simulink model "ekf9mlf_example"  (R2014a)
settings: Solver=FixedStepDiscrete  StartTime=0  StopTime=200  RelTol=1e-3
settings Model: Creator=gcampa  LastModifiedBy=gcampa
settings DataIOCC: LimitDataPoints=off  SignalLoggingSaveFormat=ModelDataLogs  SaveOutput=off  SaveTime=off
settings OptimizationCC: BlockReduction=off  BooleanDataType=off  ExpressionDepthLimit=2147483647  InitFltsAndDblsToZero=on
settings DebuggingCC: SaveWithParameterizedLinksMsg=none  UnderspecifiedInitializationDetection=Classic  SignalResolutionControl=TryResolveAllWithWarning  SolverPrmCheckMsg=none  MultiTaskDSMMsg=warning  MultiTaskCondExecSysMsg=none  FcnCallInpInsideContextMsg=UseLocalSettings  StateNameClashWarn=warning
settings HardwareCC: TargetLongLongMode=on  TargetIntDivRoundTo=Zero  TargetEndianess=LittleEndian  TargetHWDeviceType=MATLAB Host  ProdEqTarget=off
settings RTWCC: IncludeERTFirstTime=on  RTWCompilerOptimization=On
settings GRTTargetCC: TargetFcnLib=ansi_tfl_tmw.mat  CombineOutputUpdateFcns=off  GRTInterface=on

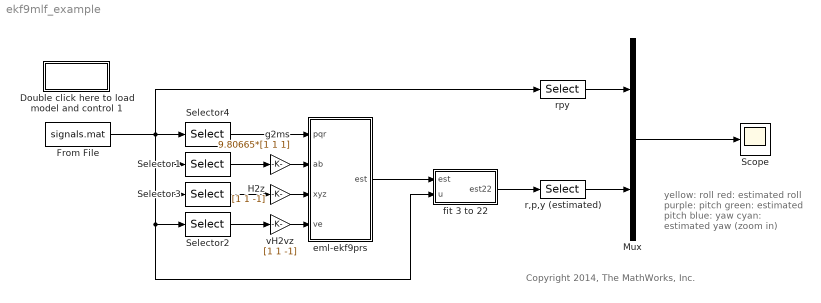
== system ekf9mlf_example ==
  note: yellow: roll
      | red: estimated roll
      | purple: pitch
      | green: estimated pitch
      | blue: yaw
      | cyan: estimated yaw
      | (zoom in)
  note: Copyright 2014, The MathWorks, Inc.
  Double click here to load model and control 1 : Subsystem
      mask Display: disp('Measured \nSignals')
  From File : FromFile  FileName=signals.mat  SampleTime=0.05
  H2z : Gain  Gain=[1 1 -1]  SaturateOnIntegerOverflow=on  OutDataTypeStr=Inherit: Same as input  ParamDataTypeStr=Inherit: Same as input
  Mux : Mux  Inputs=[3 3]
  Scope : Scope
  Selector1 : Selector  InputPortWidth=22  Indices=16:18
  Selector2 : Selector  InputPortWidth=22  Indices=13:15
  Selector3 : Selector  InputPortWidth=22  Indices=13:15
  Selector4 : Selector  InputPortWidth=22  Indices=[4:6]
  eml-ekf9prs : MATLAB Function  TreatAsAtomicUnit=on
  fit 3 to 22 : Subsystem
  g2ms : Gain  Gain=9.80665*[1 1 1]  SaturateOnIntegerOverflow=on  OutDataTypeStr=Inherit: Same as input  ParamDataTypeStr=Inherit: Same as input
  r,p,y (estimated) : Selector  InputPortWidth=22  Indices=[9 8 7]
  rpy : Selector  InputPortWidth=22  Indices=[9 8 7]
  vH2vz : Gain  Gain=[1 1 -1]  SaturateOnIntegerOverflow=on  OutDataTypeStr=Inherit: Same as input  ParamDataTypeStr=Inherit: Same as input
  wires:
  fit 3 to 22/1(est22) -> r,p,y (estimated)/1
  Selector3/1 -> H2z/1
  Selector1/1 -> g2ms/1
  g2ms/1 -> eml-ekf9prs/2(ab)
  Selector4/1 -> eml-ekf9prs/1(pqr)
  From File/1 -> rpy/1, Selector3/1, Selector2/1, fit 3 to 22/2(u), Selector1/1, Selector4/1
  eml-ekf9prs/1(est) -> fit 3 to 22/1(est)
  H2z/1 -> eml-ekf9prs/3(xyz)
  vH2vz/1 -> eml-ekf9prs/4(ve)
  Selector2/1 -> vH2vz/1
  rpy/1 -> Mux/1
  r,p,y (estimated)/1 -> Mux/2
  Mux/1 -> Scope/1

== system ekf9mlf_example/Double click here to load model and control 1 ==
  note: More information on the aircraft model and controllers can be found here:
      | http://www.mathworks.com/matlabcentral/fileexchange/3019-airlib
  note: An aircraft model in closed loop with an inner and outer loop feedback
      | linearization control system was used to generate attitude (roll, pitch and yaw)
      | as well as all the other relevant signals
  note: x:
      |
      | 01    v           (m/s)
      | 02    alpha    (rad)
      | 03    beta      (rad)
      | 04    p           (rad/s)
      | 05    q           (rad/s)
      | 06    r            (rad/s)
      | 07    psi         (rad)
      | 08    theta     (rad)
      | 09    phi        (rad)
      | 10    x           (m)
      | 11    y           (m)
      | 12    H          (m)
      |
      | x_dot (NED earth frame):
      |
      | 13    x_dot     (m/s)
      | 14    y_dot     (m/s)
      | 15    z_dot     (m/s)
      |
      | accelerations:
      |
      | 16    Ax     (g)
      | 17    Ay     (g)
      | 18    Az     (g)
      |
      | controls:
      |
      | 19    delta elevators    (rad)
      | 20    delta ailerons      (rad)
      | 21    delta rudder        (rad)
      | 22    throttle             (Fx, N)

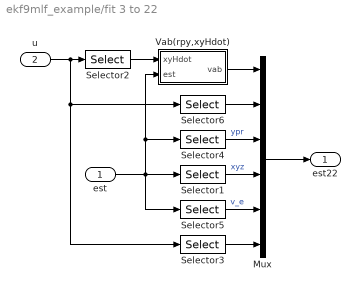
== system ekf9mlf_example/fit 3 to 22 ==
  est : Inport
  u : Inport  Port=2
  Mux : Mux  Inputs=[3 3 3 3 3 7]
  Selector1 : Selector  InputPortWidth=9  Indices=1:3
  Selector2 : Selector  InputPortWidth=22  Indices=13:15
  Selector3 : Selector  InputPortWidth=22  Indices=16:22
  Selector4 : Selector  InputPortWidth=9  Indices=[9 8 7]
  Selector5 : Selector  InputPortWidth=9  Indices=4:6
  Selector6 : Selector  InputPortWidth=22  Indices=4:6
  Vab(rpy,xyHdot) : Subsystem
  est22 : Outport
  wires:
  Selector6/1 -> Mux/2
  Selector5/1 -> Mux/5  "v_e"
  Selector1/1 -> Mux/4  "xyz"
  Selector4/1 -> Mux/3  "ypr"
  Selector3/1 -> Mux/6
  Selector2/1 -> Vab(rpy,xyHdot)/1(xyHdot)
  Vab(rpy,xyHdot)/1(vab) -> Mux/1
  u/1 -> Selector6/1, Selector3/1, Selector2/1
  est/1 -> Selector5/1, Selector4/1, Vab(rpy,xyHdot)/2(est), Selector1/1
  Mux/1 -> est22/1

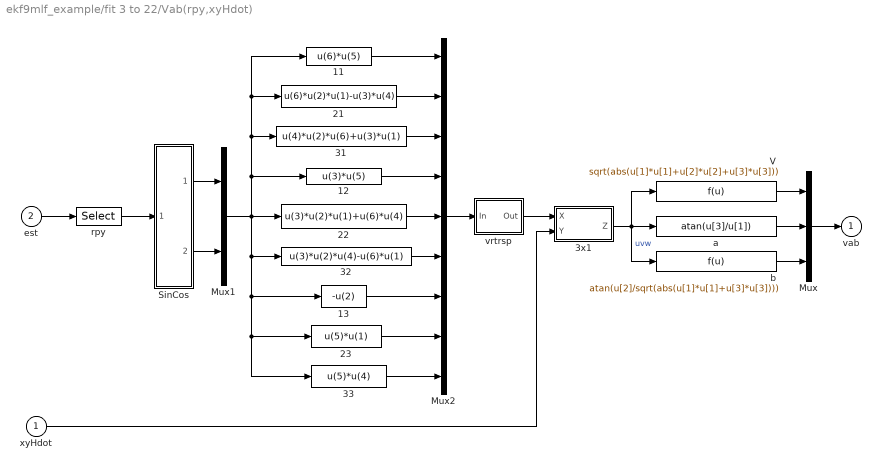
== system ekf9mlf_example/fit 3 to 22/Vab(rpy,xyHdot) ==
  xyHdot : Inport
  est : Inport  Port=2
  11 : Fcn  Expr=u(6)*u(5)
  12 : Fcn  Expr=u(3)*u(5)
  13 : Fcn  Expr=-u(2)
  21 : Fcn  Expr=u(6)*u(2)*u(1)-u(3)*u(4)
  22 : Fcn  Expr=u(3)*u(2)*u(1)+u(6)*u(4)
  23 : Fcn  Expr=u(5)*u(1)
  31 : Fcn  Expr=u(4)*u(2)*u(6)+u(3)*u(1)
  32 : Fcn  Expr=u(3)*u(2)*u(4)-u(6)*u(1)
  33 : Fcn  Expr=u(5)*u(4)
  3x1 : Subsystem  mask(3x3 Matrix Multiplication){}
      mask help:
      | Input 1   : elements of matrix X (3 by 3)
      |   Input 2   : elements of matrix Y (3 by 3)
      |   Output   : elements of matrix X*Y (3 by 3)
      mask Help:
      | <p>
      | Elements of input and output matrices are taken columnwise.
      | </p>
      mask Display: disp('Z=X*Y')
  Mux : Mux  Inputs=3
  Mux1 : Mux  Inputs=2
  Mux2 : Mux  Inputs=9
  SinCos : Subsystem  mask(SinCos){}
      mask help: Compute the sine and cosine of input, u. u is in radians.
      mask Help: web(asbhelp);
      mask Display:
      | port_label('output',1,'sin(u)','texmode','on');
      | port_label('output',2,'cos(u)','texmode','on');
  V : Fcn  Expr=sqrt(abs(u[1]*u[1]+u[2]*u[2]+u[3]*u[3]))
  a : Fcn  Expr=atan(u[3]/u[1])
  b : Fcn  Expr=atan(u[2]/sqrt(abs(u[1]*u[1]+u[3]*u[3])))
  rpy : Selector  InputPortWidth=9  Indices=7:9
  vrtrsp : Subsystem  mask(Simulink Matrix Library Block){dims=[3 3]}
      mask prompts: dims "[n m]"
      mask help:
      | Real Varying Matrix Transposition
      |   Input      : elements of matrix X (n by m)
      |   Output   : elements of matrix X' (m by n)
      mask Help:
      | <p>
      | Elements of input and output matrices are taken columnwise.
      | </p>
      | <p>
      | To use this block you should have the smxl library in your path.
      | </p>
      mask Display: disp('Y=X''')
  vab : Outport
  wires:
  rpy/1 -> SinCos/1(theta)
  vrtrsp/1(Out) -> 3x1/1(X)
  33/1 -> Mux2/9
  23/1 -> Mux2/8
  13/1 -> Mux2/7
  32/1 -> Mux2/6
  22/1 -> Mux2/5
  12/1 -> Mux2/4
  31/1 -> Mux2/3
  21/1 -> Mux2/2
  11/1 -> Mux2/1
  SinCos/1(sin(theta)) -> Mux1/1
  SinCos/2(cos(theta)) -> Mux1/2
  Mux1/1 -> 22/1, 11/1, 21/1, 31/1, 12/1, 32/1, 13/1, 23/1, 33/1
  Mux2/1 -> vrtrsp/1(In)
  xyHdot/1 -> 3x1/2(Y)
  b/1 -> Mux/3
  V/1 -> Mux/1
  a/1 -> Mux/2
  Mux/1 -> vab/1
  3x1/1(Z) -> b/1, a/1, V/1  "uvw"
  est/1 -> rpy/1

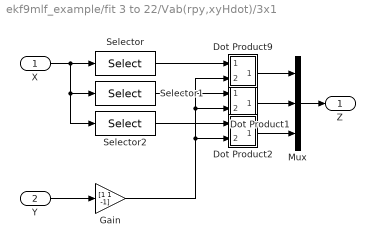
== system ekf9mlf_example/fit 3 to 22/Vab(rpy,xyHdot)/3x1 ==
  X : Inport
  Y : Inport  Port=2
  Dot Product1 : Subsystem  mask(Dot Product){}
      mask help:
      | Inner (dot) product.
      | y = sum(conj(u1).*u2). The operand u1 corresponds to the top (or left) input port.
      mask init:
      | t=(0:.1:2*pi)';
      | x=cos(t);
      | y=sin(t);
      | r=0.05;
      mask Help: Computes the inner (dot) product of the inputs: sum(u1.*u2).  The inputs are vectors of the same length. Output is a scalar.
      mask Display: patch([x*r+0.5],[y*r+0.5])
  Dot Product2 : Subsystem  mask(Dot Product){}
      mask help:
      | Inner (dot) product.
      | y = sum(conj(u1).*u2). The operand u1 corresponds to the top (or left) input port.
      mask init:
      | t=(0:.1:2*pi)';
      | x=cos(t);
      | y=sin(t);
      | r=0.05;
      mask Help: Computes the inner (dot) product of the inputs: sum(u1.*u2).  The inputs are vectors of the same length. Output is a scalar.
      mask Display: patch([x*r+0.5],[y*r+0.5])
  Dot Product9 : Subsystem  mask(Dot Product){}
      mask help:
      | Inner (dot) product.
      | y = sum(conj(u1).*u2). The operand u1 corresponds to the top (or left) input port.
      mask init:
      | t=(0:.1:2*pi)';
      | x=cos(t);
      | y=sin(t);
      | r=0.05;
      mask Help: Computes the inner (dot) product of the inputs: sum(u1.*u2).  The inputs are vectors of the same length. Output is a scalar.
      mask Display: patch([x*r+0.5],[y*r+0.5])
  Gain : Gain  Gain=[1 1 -1]  OutDataTypeStr=Inherit: Same as input  ParamDataTypeStr=Inherit: Same as input
  Mux : Mux  Inputs=3
  Selector : Selector  InputPortWidth=9  Indices=[1:3]
  Selector1 : Selector  InputPortWidth=9  Indices=[4:6]
  Selector2 : Selector  InputPortWidth=9  Indices=[7:9]
  Z : Outport
  wires:
  Mux/1 -> Z/1
  Gain/1 -> Dot Product9/2(In2), Dot Product1/2(In2), Dot Product2/2(In2)
  Y/1 -> Gain/1
  Dot Product2/1(Out1) -> Mux/3
  Selector2/1 -> Dot Product2/1(In1)
  Selector1/1 -> Dot Product1/1(In1)
  Dot Product1/1(Out1) -> Mux/2
  Dot Product9/1(Out1) -> Mux/1
  Selector/1 -> Dot Product9/1(In1)
  X/1 -> Selector2/1, Selector1/1, Selector/1

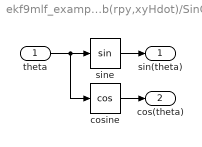
== system ekf9mlf_example/fit 3 to 22/Vab(rpy,xyHdot)/SinCos ==
  theta : Inport
  cosine : Trigonometry  Operator=cos
  sine : Trigonometry
  sin(theta) : Outport
  cos(theta) : Outport  Port=2
  wires:
  cosine/1 -> cos(theta)/1
  sine/1 -> sin(theta)/1
  theta/1 -> cosine/1, sine/1

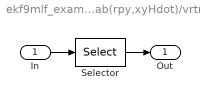
== system ekf9mlf_example/fit 3 to 22/Vab(rpy,xyHdot)/vrtrsp ==
  In : Inport
  Selector : Selector  InputPortWidth=dims(1)*dims(2)  Indices=reshape(reshape(1:dims(1)*dims(2),dims(1),dims(2))',dims(1)*dims(2),1)
  Out : Outport
  wires:
  In/1 -> Selector/1
  Selector/1 -> Out/1

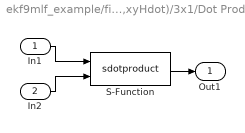
== system ekf9mlf_example/fit 3 to 22/Vab(rpy,xyHdot)/3x1/Dot Product1 ==
  In1 : Inport
  In2 : Inport  Port=2
  S-Function : S-Function  FunctionName=sdotproduct  EnableBusSupport=off
  Out1 : Outport
  wires:
  In2/1 -> S-Function/2
  In1/1 -> S-Function/1
  S-Function/1 -> Out1/1

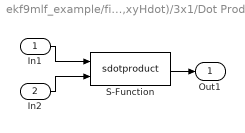
== system ekf9mlf_example/fit 3 to 22/Vab(rpy,xyHdot)/3x1/Dot Product2 ==
  In1 : Inport
  In2 : Inport  Port=2
  S-Function : S-Function  FunctionName=sdotproduct  EnableBusSupport=off
  Out1 : Outport
  wires:
  S-Function/1 -> Out1/1
  In1/1 -> S-Function/1
  In2/1 -> S-Function/2

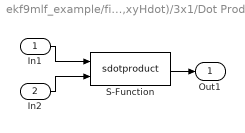
== system ekf9mlf_example/fit 3 to 22/Vab(rpy,xyHdot)/3x1/Dot Product9 ==
  In1 : Inport
  In2 : Inport  Port=2
  S-Function : S-Function  FunctionName=sdotproduct  EnableBusSupport=off
  Out1 : Outport
  wires:
  S-Function/1 -> Out1/1
  In1/1 -> S-Function/1
  In2/1 -> S-Function/2

== matlab function ekf9mlf_example/eml-ekf9prs ==
  data: pqr input; ab input; xyz input; ve input; est output; T parameter
function est=ekf9prs(pqr,ab,xyz,ve,T)

%% initialization

% constants
W=1e-3*eye(9);  % state noise covariance
V=0.1*eye(6);   % output noise covariance
Plim=1e-5;      % P limiter

% state variables
persistent P x
if isempty(P) || isempty(x),
    P=zeros(9);
    x=[0 0 60 60*cos(0) 60*sin(0) 60*sin(-0.03) 0 -0.03 0]'; % initial state
end

%% the output is the previous state.

est = x;

%% Calculate next state

% define dimensions
nx=9;nu=6;ny=6;

% states
phi=x(7);
theta=x(8);
psi=x(9);

% inputs
ax=ab(1);
ay=ab(2);
az=ab(3);
p=pqr(1);
q=pqr(2);
r=pqr(3);

% measured state
y=[xyz(:);ve(:)];

% x propagation:
g=[0 0 9.80665]';

% body to earth frame
Toc=transpose([cos(psi) sin(psi) 0; -sin(psi) cos(psi) 0; 0 0 1]);
Tcf=transpose([cos(theta) 0 -sin(theta); 0 1 0; sin(theta) 0 cos(theta)]);
Tfb=transpose([1 0 0; 0 cos(phi) sin(phi); 0 -sin(phi) cos(phi)]);
Teb=Toc*Tcf*Tfb;

% omega to attitude dot
Taw=transpose([1 0 0; sin(phi)*tan(theta) cos(phi) sin(phi)/cos(theta); cos(phi)*tan(theta) -sin(phi) cos(phi)/cos(theta)]);

% equations
pdot=x(4:6);
vdot=g+Teb*[ax;ay;az];
adot=Taw*[p;q;r];
xdot=[pdot;vdot;adot];

% propagation:
xm=x+T*xdot;

% A matrix
a81 = [                                                                                                                                0
    0
    0
    0
    0
    0
    0
    0
    0
    0
    0
    0
    0
    0
    0
    0
    0
    0
    0
    0
    0
    0
    0
    0
    0
    0
    0
    1
    0
    0
    0
    0
    0
    0
    0
    0
    0
    1
    0
    0
    0
    0
    0
    0
    0
    0
    0
    1
    0
    0
    0
    0
    0
    0
    0
    0
    0
    (sin(psi)*sin(phi)+cos(psi)*sin(theta)*cos(phi))*ay+(sin(psi)*cos(phi)-cos(psi)*sin(theta)*sin(phi))*az
    (-cos(psi)*sin(phi)+sin(psi)*sin(theta)*cos(phi))*ay+(-cos(psi)*cos(phi)-sin(psi)*sin(theta)*sin(phi))*az
    cos(theta)*cos(phi)*ay-cos(theta)*sin(phi)*az
    cos(phi)*tan(theta)*q-sin(phi)*tan(theta)*r
    -sin(phi)*q-cos(phi)*r
    cos(phi)/cos(theta)*q-sin(phi)/cos(theta)*r
    0
    0
    0
    -cos(psi)*sin(theta)*ax+cos(psi)*cos(theta)*sin(phi)*ay+cos(psi)*cos(theta)*cos(phi)*az
    -sin(psi)*sin(theta)*ax+sin(psi)*cos(theta)*sin(phi)*ay+sin(psi)*cos(theta)*cos(phi)*az
    -cos(theta)*ax-sin(theta)*sin(phi)*ay-sin(theta)*cos(phi)*az
    sin(phi)*(1+tan(theta)^2)*q+cos(phi)*(1+tan(theta)^2)*r
    0
    sin(phi)/cos(theta)^2*q*sin(theta)+cos(phi)/cos(theta)^2*r*sin(theta)
    0
    0
    0
    -sin(psi)*cos(theta)*ax+(-cos(psi)*cos(phi)-sin(psi)*sin(theta)*sin(phi))*ay+(cos(psi)*sin(phi)-sin(psi)*sin(theta)*cos(phi))*az
    cos(psi)*cos(theta)*ax+(-sin(psi)*cos(phi)+cos(psi)*sin(theta)*sin(phi))*ay+(sin(psi)*sin(phi)+cos(psi)*sin(theta)*cos(phi))*az
    0
    0
    0
    0
    ];

a=reshape(a81,nx,nx);
C = eye(ny,nx);

% euler forward step
A = eye(size(a))+T*a; 

% store eigenvalues
% global eiga
% eiga=[eiga eig(a)];
%%plot(eiga','.');sgrid

% perfect sample and hold
% A = expm(a*T);

% tustin
% alpha=2/T;invterm = inv(eye(nx)-(1/alpha)*a);
% A = (eye(nx) + (1/alpha)*a)*invterm;

% find K
Pm=W+A*P*A';
K=Pm*C'*inv(V+C*Pm*C');

% EKF update equations
Pp=(eye(size(Pm))-K*C)*Pm;
xp=xm+K*(y-C*xm);

% psi limiter
xp(9)=mod(xp(9)+pi,2*pi)-pi;

% alternative Joseph form to retain symmetry
% Pp=(eye(size(Pm))-K*C)*Pm*(eye(size(Pm))-K*C)'+K*V*K';

% ball norm limiter
nrm=sqrt(Pp(:)'*Pp(:));
Pp=Pp*min(nrm,Plim)/max(nrm,realmin);

% store state
x=xp;
P=Pp;
